simulink model "power_sixpulses"  (Simulink 6.0)
settings: Solver=ode23s  SolverMode=SingleTasking  StartTime=0.0  StopTime=0.035  RelTol=1e-5  AbsTol=1e-5
libraries: powerlib x12, powerlib_extras x1
settings Model: Creator=sybille  LastModifiedBy=batserve  ExtModeTrigMode=oneshot  ExtModeArmWhenConnect=off  ExtModeAutoUpdateStatusClock=off
settings SolverCC: MaxOrder=1
settings DataIOCC: LimitDataPoints=off  SaveOutput=off  SaveTime=off  SignalLoggingName=sigsOut
settings OptimizationCC: BlockReduction=off  BooleanDataType=off
settings DebuggingCC: SolverPrmCheckMsg=none  UnconnectedInputMsg=none  UnconnectedOutputMsg=none  UnconnectedLineMsg=none
settings HardwareCC: TargetUnknown=on
settings RTWCC: TemplateMakefile=grt_unix.tmf

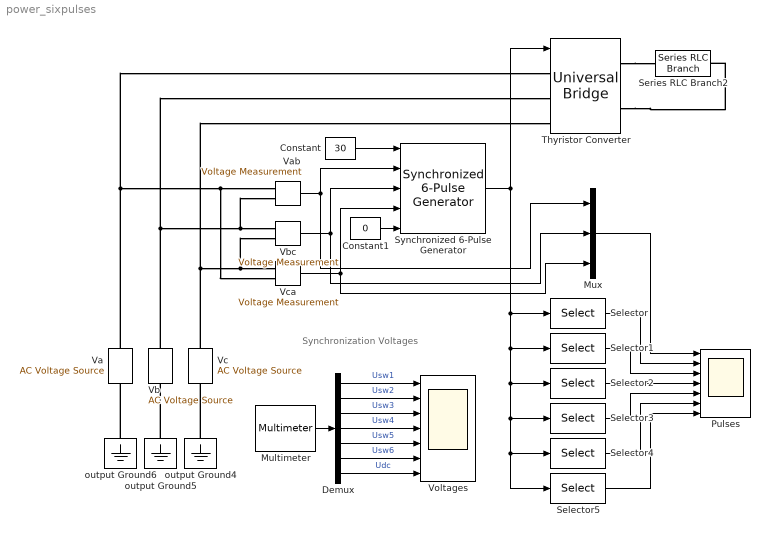
== system power_sixpulses ==
  note: Synchronization Voltages
  Constant : Constant  Value=30
  Constant1 : Constant  Value=0
  Demux : Demux  Outputs=7
  Multimeter : powerlib/Measurements/Multimeter  Tag=PoWeRsYsTeMmEaSuReMeNt  PhasorSimulation=off  OutputType=Magnitude  sel=[1 2 3 4 5 6 10]  L=16  Gain=[-1 -1 -1 -1 -1 -1 1]  yselected={'Usw1: Thyristor Converter','Usw2: Thyristor Converter','Usw3: Thyristor Converter','Usw4: Thyristor Converter','Usw5: Thyristor Converter','Usw6: Thyristor Converter','Udc: Thyristor Converter'};  PSBOutputType=1  PSBequivalent=0  AxesSetting=[0,0.1,-100,100]  Display=0  SavedBlockNames=-11
      settings: AttributesFormatString=\n
  Mux : Mux  Inputs=3
  Pulses : Scope  NumInputPorts=7
      settings: TimeRange=0.035  YMin=-400~-1~-1~-1~0~0~0  YMax=400~1~1~1~1~1~1  SaveName=VI_scope  SampleInput=on  SampleTime=1/60/512
  Selector : Selector  InputPortWidth=6
  Selector1 : Selector  Elements=2  InputPortWidth=6
  Selector2 : Selector  Elements=3  InputPortWidth=6
  Selector3 : Selector  Elements=4  InputPortWidth=6
  Selector4 : Selector  Elements=5  InputPortWidth=6
  Selector5 : Selector  Elements=6  InputPortWidth=6
  Series RLC Branch2 : powerlib/Elements/Series RLC Branch  PhysicalDomain=powersysdomain  SubClassName=unknown  PortType=p1  LConnTagsString=__new0  RConnTagsString=__new0  Resistance=2  Inductance=0  Capacitance=inf  Measurements=None
  Synchronized 6-Pulse Generator : powerlib_extras/Control  Blocks/Synchronized 6-Pulse Generator  freq=60  pwidth=10  Double_Pulse=on
  Thyristor Converter : powerlib/Power Electronics/Universal Bridge  Arms=3  SnubberResistance=500  SnubberCapacitance=1e-6  Device=Thyristors  Ron=1e-3  Lon=0  ForwardVoltages="[  0.8  0.8  ]"  ForwardVoltage=0  GTOparameters=[ 10e-6 , 20e-6 ]  IGBTparameters=[ 1e-6 , 2e-6 ]  Measurements=All voltages and currents
  Va : powerlib/Electrical Sources/AC Voltage Source  Description=source block  Orientation=up  Amplitude=200  Phase=0  Frequency=60  SampleTime=0  Measurements=None
      settings: AttributesFormatString=\n
  Vab : powerlib/Measurements/Voltage Measurement  Tag=PoWeRsYsTeMmEaSuReMeNt  PhasorSimulation=off  OutputType=Magnitude  PSBequivalent=0
  Vb : powerlib/Electrical Sources/AC Voltage Source  Description=source block  Orientation=up  Amplitude=200  Phase=-120  Frequency=60  SampleTime=0  Measurements=None
      settings: AttributesFormatString=\n
  Vbc : powerlib/Measurements/Voltage Measurement  Tag=PoWeRsYsTeMmEaSuReMeNt  PhasorSimulation=off  OutputType=Magnitude  PSBequivalent=0
  Vc : powerlib/Electrical Sources/AC Voltage Source  Description=source block  Orientation=up  Amplitude=200  Phase=120  Frequency=60  SampleTime=0  Measurements=None
      settings: AttributesFormatString=\n
  Vca : powerlib/Measurements/Voltage Measurement  Tag=PoWeRsYsTeMmEaSuReMeNt  PhasorSimulation=off  OutputType=Magnitude  PSBequivalent=0
  Voltages : Scope  NumInputPorts=7
      settings: TimeRange=0.035  YMin=-400~-1~-1~-1~0~0~0  YMax=400~1~1~1~1~1~1  SaveName=VI_scope1  SampleInput=on  SampleTime=1/60/512
  output Ground4 : powerlib/Elements/Ground  Orientation=down  PhysicalDomain=powersysdomain  SubClassName=unknown  PortType=p1  LConnTagsString=a
  output Ground5 : powerlib/Elements/Ground  Orientation=down  PhysicalDomain=powersysdomain  SubClassName=unknown  PortType=p1  LConnTagsString=a
  output Ground6 : powerlib/Elements/Ground  Orientation=down  PhysicalDomain=powersysdomain  SubClassName=unknown  PortType=p1  LConnTagsString=a
  wires:
  Constant/1 -> Synchronized 6-Pulse Generator/1
  Selector5/1 -> Pulses/7
  Selector4/1 -> Pulses/6
  Selector3/1 -> Pulses/5
  Selector2/1 -> Pulses/4
  Selector1/1 -> Pulses/3
  Selector/1 -> Pulses/2
  Mux/1 -> Pulses/1
  Constant1/1 -> Synchronized 6-Pulse Generator/5
  Vca/1 -> Synchronized 6-Pulse Generator/4, Mux/3
  Vbc/1 -> Synchronized 6-Pulse Generator/3, Mux/2
  Vab/1 -> Synchronized 6-Pulse Generator/2, Mux/1
  Synchronized 6-Pulse Generator/1 -> Selector/1, Selector1/1, Selector2/1, Selector3/1, Selector4/1, Selector5/1, Thyristor Converter/1
  Multimeter/1 -> Demux/1
  Demux/1 -> Voltages/1  "Usw1"
  Demux/2 -> Voltages/2  "Usw2"
  Demux/3 -> Voltages/3  "Usw3"
  Demux/4 -> Voltages/4  "Usw4"
  Demux/5 -> Voltages/5  "Usw5"
  Demux/6 -> Voltages/6  "Usw6"
  Demux/7 -> Voltages/7  "Udc"
  connections:
  Thyristor Converter/RConn1 -- Series RLC Branch2/LConn1
  output Ground6/LConn1 -- Va/LConn1
  output Ground5/LConn1 -- Vb/LConn1
  output Ground4/LConn1 -- Vc/LConn1
  Thyristor Converter/RConn2 -- Series RLC Branch2/RConn1
  Vb/RConn1 -- Vbc/LConn1 -- Vab/LConn2 -- Thyristor Converter/LConn2
  Vc/RConn1 -- Vca/LConn1 -- Vbc/LConn2 -- Thyristor Converter/LConn3
  Va/RConn1 -- Vab/LConn1 -- Vca/LConn2 -- Thyristor Converter/LConn1
